simulink model "five_kw_wind_turbine_design"  (R2014b)
settings: Solver=ode45  StartTime=0.0  StopTime=2  RelTol=1e-3
settings Model: Creator=Amr Saleh  LastModifiedBy=Amr Saleh

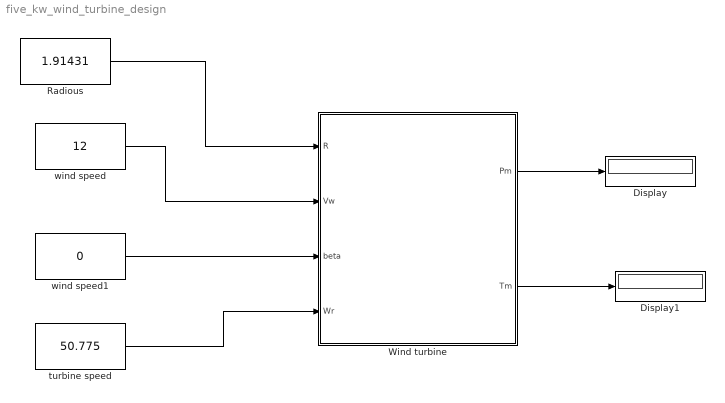
== system five_kw_wind_turbine_design ==
  Display : Display
  Display1 : Display
  Radious : Constant  Value=1.91431
  Wind turbine : Subsystem
  turbine speed : Constant  Value=50.775
  wind speed : Constant  Value=12
  wind speed1 : Constant  Value=0
  wires:
  Radious/1 -> Wind turbine/1(R)
  wind speed/1 -> Wind turbine/2(Vw)
  wind speed1/1 -> Wind turbine/3(beta)
  turbine speed/1 -> Wind turbine/4(Wr)
  Wind turbine/1(Pm) -> Display/1
  Wind turbine/2(Tm) -> Display1/1

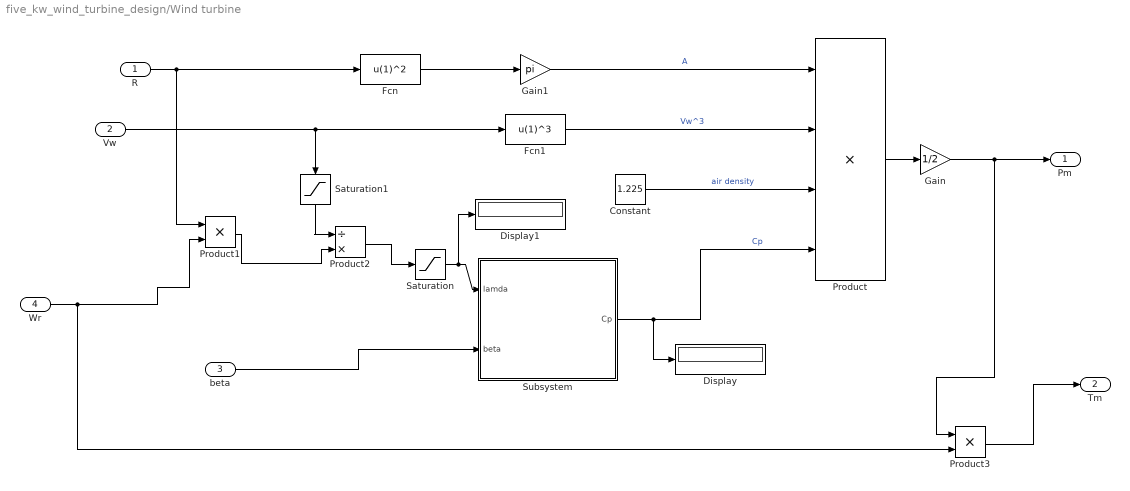
== system five_kw_wind_turbine_design/Wind turbine ==
  R : Inport
  Vw : Inport  Port=2
  beta : Inport  Port=3
  Wr : Inport  Port=4
  Constant : Constant  Value=1.225
  Display : Display
  Display1 : Display
  Fcn : Fcn  Expr=u(1)^2
  Fcn1 : Fcn  Expr=u(1)^3
  Gain : Gain  Gain=1/2
  Gain1 : Gain  Gain=pi
  Product : Product  Inputs=4
  Product1 : Product
  Product2 : Product  Inputs=/*
  Product3 : Product
  Saturation : Saturate  UpperLimit=inf  LowerLimit=1e-6
  Saturation1 : Saturate  UpperLimit=inf  LowerLimit=1e-6
  Subsystem : Subsystem
  Pm : Outport
  Tm : Outport  Port=2
  wires:
  Gain1/1 -> Product/1  "A"
  Fcn1/1 -> Product/2  "Vw^3"
  Constant/1 -> Product/3  "air density"
  Subsystem/1(Cp) -> Display/1, Product/4  "Cp"
  Gain/1 -> Product3/1, Pm/1
  Product/1 -> Gain/1
  Fcn/1 -> Gain1/1
  R/1 -> Fcn/1, Product1/1
  Vw/1 -> Fcn1/1, Saturation1/1
  beta/1 -> Subsystem/2(beta)
  Wr/1 -> Product3/2, Product1/2
  Product1/1 -> Product2/2
  Product2/1 -> Saturation/1
  Saturation/1 -> Display1/1, Subsystem/1(lamda)
  Saturation1/1 -> Product2/1
  Product3/1 -> Tm/1

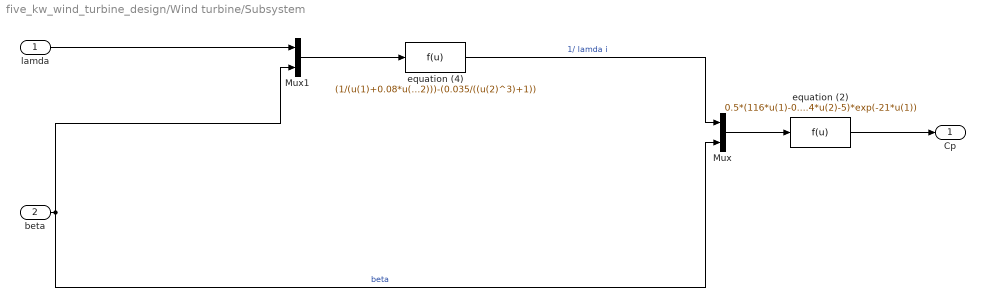
== system five_kw_wind_turbine_design/Wind turbine/Subsystem ==
  lamda : Inport
  beta : Inport  Port=2
  Mux : Mux  Inputs=2
  Mux1 : Mux  Inputs=2
  equation (2) : Fcn  Expr=0.5*(116*u(1)-0.4*u(2)-5)*exp(-21*u(1))
  equation (4) : Fcn  Expr=(1/(u(1)+0.08*u(2)))-(0.035/((u(2)^3)+1))
  Cp : Outport
  wires:
  equation (2)/1 -> Cp/1
  Mux/1 -> equation (2)/1
  equation (4)/1 -> Mux/1  "1/ lamda i"
  beta/1 -> Mux/2, Mux1/2  "beta"
  Mux1/1 -> equation (4)/1
  lamda/1 -> Mux1/1
